simulink model "SSI_Simulator"  (R2020a)
settings: Solver=VariableStepAuto  StartTime=0.0  StopTime=10  RelTol=1e-3
values from neighbouring files (symbols this model uses):
  D = 60    [para.m]    (also in parameter.m)
  E0 = 100    [para.m]    (also in parameter.m)
  Kgov = 2    [para.m]    (also in parameter.m)
  Ki = 0.5    [para.m]    (also in parameter.m)
  Kp = 0    [para.m]    (also in parameter.m)
  KQ = 0.05    [para.m]    (also in parameter.m)
  Kvq = 1    [para.m]    (also in parameter.m)
  M = 1    [para.m]    (also in parameter.m)
  Pm = 300    [para.m]    (also in parameter.m)
  Qref = 0    [para.m]    (also in parameter.m)
  Qsig = 1    [para.m]    (also in parameter.m)
  Tgov = 0.1    [para.m]    (also in parameter.m)
  Tvq = 0.001    [para.m]    (also in parameter.m)
  Vl = 100    [para.m]    (also in parameter.m)
  Vref = 100    [para.m]    (also in parameter.m)
  wref = 2 * pi * 60    (= 376.991118431)    [para.m]    (also in parameter.m)
  Y1 = complex(G1, B1)    [para.m]    (also in parameter.m)
  Y2 = complex(G2 ,B2)    [para.m]    (also in parameter.m)
  Yg = 0    [para.m]    (also in parameter.m)
  YGG = inv(Y1 + Y2 + Yg)    [para.m]    (also in parameter.m)
undefined symbols (not defined in the file or in its folder): sw
libraries: simulink x1
settings Model: Creator=EPESL  LastModifiedBy=EPESL
settings DataIOCC: ReturnWorkspaceOutputs=off
settings DebuggingCC: AlgebraicLoopMsg=none  ArithmeticOperatorsInVariantConditions=warning
settings SFSimCC: CustomCodeUndefinedFunction=UseInterfaceOnly

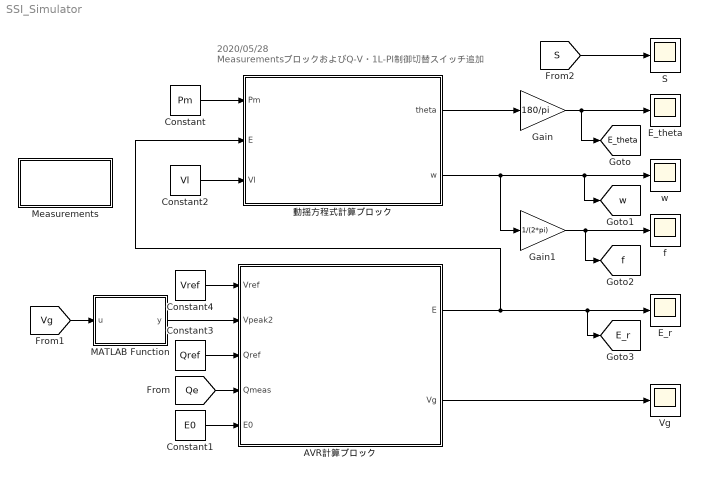
== system SSI_Simulator ==
  note: 2020/05/28
      | MeasurementsブロックおよびQ-V・1L-PI制御切替スイッチ追加
  AVR計算ブロック : Subsystem
  Constant : Constant  Value=Pm
  Constant1 : Constant  Value=E0
  Constant2 : Constant  Value=Vl
  Constant3 : Constant  Value=Qref
  Constant4 : Constant  Value=Vref
  E_r : Scope
  E_theta : Scope
  Gain : Gain  Gain=180/pi
  Gain1 : Gain  Gain=1/(2*pi)
  MATLAB Function : MATLAB Function  TreatAsAtomicUnit=on
  Measurements : Subsystem
      mask Display: color('blue');disp('Measurements')
  S : Scope
  Vg : Scope
  f : Scope
  w : Scope
  動揺方程式計算ブロック : Subsystem
  tag scope: E_r=global, E_theta=global, f=global, w=global
  wires:
  [S] -> S/1
  AVR計算ブロック/2(Vg) -> Vg/1
  MATLAB Function/1(y) -> AVR計算ブロック/2(Vpeak2)
  Constant3/1 -> AVR計算ブロック/3(Qref)
  Constant4/1 -> AVR計算ブロック/1(Vref)
  [Qe] -> AVR計算ブロック/4(Qmeas)
  [Vg] -> MATLAB Function/1(u)
  Constant/1 -> 動揺方程式計算ブロック/1(Pm)
  Constant2/1 -> 動揺方程式計算ブロック/3(Vl)
  Gain/1 -> [E_theta], E_theta/1
  動揺方程式計算ブロック/2(w) -> Gain1/1, [w], w/1
  AVR計算ブロック/1(E) -> 動揺方程式計算ブロック/2(E), [E_r], E_r/1
  Gain1/1 -> [f], f/1
  動揺方程式計算ブロック/1(theta) -> Gain/1
  Constant1/1 -> AVR計算ブロック/5(E0)

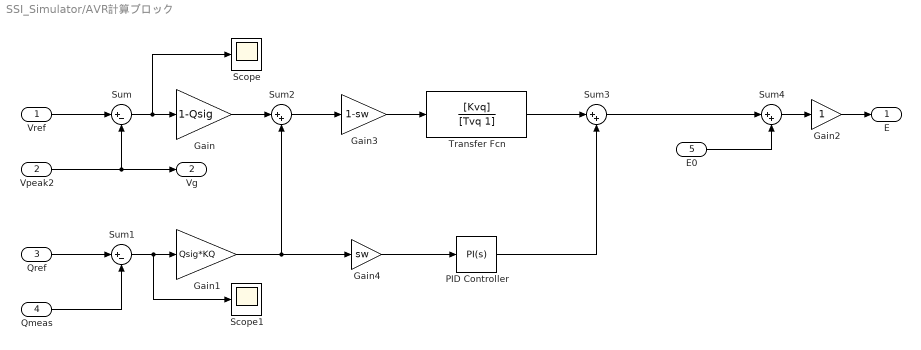
== system SSI_Simulator/AVR計算ブロック ==
  Vref : Inport
  Vpeak2 : Inport  Port=2
  Qref : Inport  Port=3
  Qmeas : Inport  Port=4
  E0 : Inport  Port=5
  Gain : Gain  Gain=1-Qsig
  Gain1 : Gain  Gain=Qsig*KQ
  Gain2 : Gain
  Gain3 : Gain  Gain=1-sw
  Gain4 : Gain  Gain=sw
  PID Controller : simulink/Continuous/PID Controller  Controller=PI  Form=Parallel  TimeDomain=Continuous-time  UseExternalTs=off  SampleTime=-1  IntegratorMethod=Forward Euler  FilterMethod=Forward Euler  ControllerParametersSource=internal  P=Kp  I=Ki  D=0  UseFilter=on  N=100  TunerSelectOption=Transfer Function Based (PID Tuner App)  InitialConditionSource=internal  InitialConditionForIntegrator=0  InitialConditionForFilter=0  DifferentiatorICPrevScaledInput=0  ExternalReset=none  TrackingMode=off  Kt=1  LimitOutput=off  UpperSaturationLimit=inf  LowerSaturationLimit=-inf  LinearizeAsGain=on  AntiWindupMode=none  Kb=1  POutMin=[]  POutMax=[]  IOutMin=[]  IOutMax=[]  DOutMin=[]  DOutMax=[]  NOutMin=[]  NOutMax=[]  SumOutMin=[]  SumOutMax=[]  SaturationOutMin=[]  SaturationOutMax=[]  PParamMin=[]  PParamMax=[]  IParamMin=[]  IParamMax=[]  DParamMin=[]  DParamMax=[]  NParamMin=[]  NParamMax=[]  KbParamMin=[]  KbParamMax=[]  KtParamMin=[]  KtParamMax=[]  KbOutMin=[]  KbOutMax=[]  KtOutMin=[]  KtOutMax=[]  IntegratorOutMin=[]  IntegratorOutMax=[]  FilterOutMin=[]  FilterOutMax=[]  SumI1OutMin=[]  SumI1OutMax=[]  SumI2OutMin=[]  SumI2OutMax=[]  SumI3OutMin=[]  SumI3OutMax=[]  SumI4OutMin=[]  SumI4OutMax=[]  SumDOutMin=[]  SumDOutMax=[]  DifferentiatorOutMin=[]  DifferentiatorOutMax=[]  FilterDiffOutCoefMin=[]  FilterDiffOutCoefMax=[]  ReciprocalOutMin=[]  ReciprocalOutMax=[]  SumDenOutMin=[]  SumDenOutMax=[]  SumNumOutMin=[]  SumNumOutMax=[]  DivideOutMin=[]  DivideOutMax=[]  UdiffTsProdOutMin=[]  UdiffTsProdOutMax=[]  NTsProdOutMin=[]  NTsProdOutMax=[]  UintegralTsProdOutMin=[]  UintegralTsProdOutMax=[]  UngainTsProdOutMin=[]  UngainTsProdOutMax=[]  IntegratorContinuousStateAttributes=''  IntegratorStateMustResolveToSignalObject=off  IntegratorRTWStateStorageClass=Auto  FilterContinuousStateAttributes=''  FilterStateMustResolveToSignalObject=off  FilterRTWStateStorageClass=Auto  ParallelPVariant=InternalParameters  IdealPVariant=Disabled  IVariant=InternalParameters  DVariant=Disabled  IntegratorVariant=Continuous  SatVariant=Disabled  AWVariant=Passthrough  PCopyVariant=Disabled  TRVariant=Disabled  FdbkBlocksVariant=Forward  IdealPFdbkVariant=Disabled  SatFdbkVariant=Disabled  DerivativeFilterVariant=Disabled  NVariant=Disabled  NCopyVariant=Disabled_SignalSpec  FilterICVariant=Disabled  IntegratorICVariant=InternalICs  ExternalResetVariant=Disabled  TRSumVariant=Passthrough  SumFdbkVariant=Disabled  SumVariant=Sum_PI  TsampFilterVariant=InternalTs  TsampNgainVariant=Passthrough  TsampIntegralVariant=Passthrough
  Scope : Scope
  Scope1 : Scope
  Sum : Sum  Inputs=|+-
  Sum1 : Sum  Inputs=|+-
  Sum2 : Sum  Inputs=|++
  Sum3 : Sum  Inputs=|++
  Sum4 : Sum  Inputs=|++
  Transfer Fcn : TransferFcn  Numerator=[Kvq]  Denominator=[Tvq 1]
  E : Outport
  Vg : Outport  Port=2
  wires:
  Transfer Fcn/1 -> Sum3/1
  Sum3/1 -> Sum4/1
  Qref/1 -> Sum1/1
  Gain1/1 -> Gain4/1, Sum2/2
  Sum4/1 -> Gain2/1
  Gain2/1 -> E/1
  PID Controller/1 -> Sum3/2
  Qmeas/1 -> Sum1/2
  Vpeak2/1 -> Vg/1, Sum/2
  Sum/1 -> Scope/1, Gain/1
  Vref/1 -> Sum/1
  Gain/1 -> Sum2/1
  Sum1/1 -> Scope1/1, Gain1/1
  Sum2/1 -> Gain3/1
  Gain3/1 -> Transfer Fcn/1
  Gain4/1 -> PID Controller/1
  E0/1 -> Sum4/2

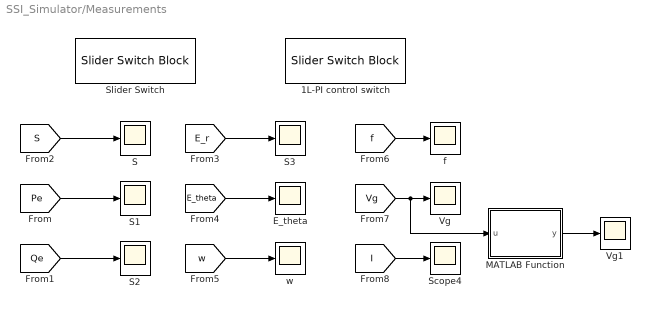
== system SSI_Simulator/Measurements ==
  1L-PI control switch : SliderSwitchBlock  LabelPosition=Hide
      settings: Values={{'1L', 'PI'}, [0 1]}
  E_theta : Scope
  MATLAB Function : MATLAB Function  TreatAsAtomicUnit=on
  S{,1..3} (4 alike) : Scope
  Scope4 : Scope
  Slider Switch : SliderSwitchBlock  LabelPosition=Hide
      settings: Values={{'Q', 'V'}, [1 0]}
  Vg : Scope
  Vg1 : Scope
  f : Scope
  w : Scope
  wires:
  [S] -> S/1
  [Pe] -> S1/1
  [Qe] -> S2/1
  [E_r] -> S3/1
  [w] -> w/1
  [I] -> Scope4/1
  [Vg] -> MATLAB Function/1(u), Vg/1
  [E_theta] -> E_theta/1
  [f] -> f/1
  MATLAB Function/1(y) -> Vg1/1

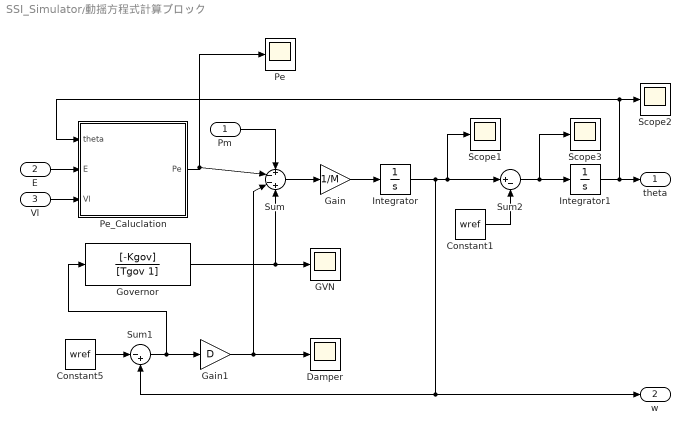
== system SSI_Simulator/動揺方程式計算ブロック ==
  Pm : Inport
  E : Inport  Port=2
  Vl : Inport  Port=3
  Constant1 : Constant  Value=wref
  Constant5 : Constant  Value=wref
  Damper : Scope
  GVN : Scope
  Gain : Gain  Gain=1/M
  Gain1 : Gain  Gain=D
  Governor : TransferFcn  Numerator=[-Kgov]  Denominator=[Tgov 1]
  Integrator : Integrator  InitialCondition=2*pi*60
  Integrator1 : Integrator
  Pe : Scope
  Pe_Caluclation : Subsystem
  Scope1 : Scope
  Scope2 : Scope
  Scope3 : Scope
  Sum : Sum  Inputs=+--+
  Sum1 : Sum  Inputs=|-+
  Sum2 : Sum  Inputs=|+-
  theta : Outport  VectorParamsAs1DForOutWhenUnconnected=off
  w : Outport  Port=2  VectorParamsAs1DForOutWhenUnconnected=off
  wires:
  Sum1/1 -> Governor/1, Gain1/1
  Gain/1 -> Integrator/1
  Constant5/1 -> Sum1/1
  Sum/1 -> Gain/1
  Gain1/1 -> Damper/1, Sum/3
  Integrator1/1 -> Pe_Caluclation/1(theta), Scope2/1, theta/1
  Pm/1 -> Sum/1
  Vl/1 -> Pe_Caluclation/3(Vl)
  Pe_Caluclation/1(Pe) -> Sum/2, Pe/1
  E/1 -> Pe_Caluclation/2(E)
  Governor/1 -> GVN/1, Sum/4
  Sum2/1 -> Scope3/1, Integrator1/1
  Integrator/1 -> Sum2/1, Scope1/1, w/1, Sum1/2
  Constant1/1 -> Sum2/2

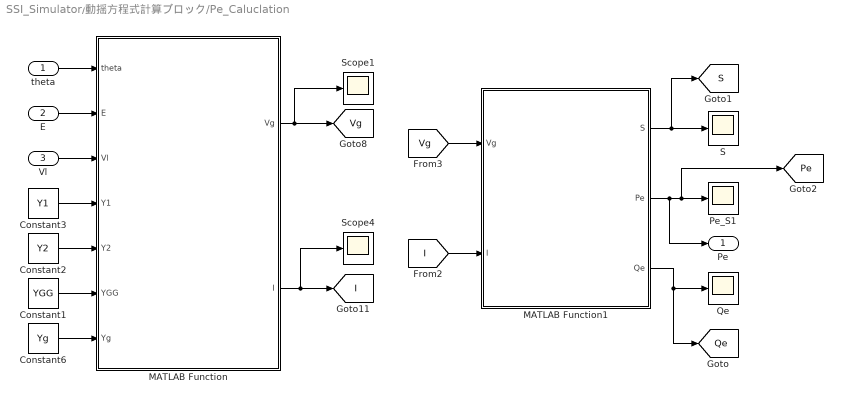
== system SSI_Simulator/動揺方程式計算ブロック/Pe_Caluclation ==
  theta : Inport
  E : Inport  Port=2
  Vl : Inport  Port=3
  Constant1 : Constant  Value=YGG
  Constant2 : Constant  Value=Y2
  Constant3 : Constant  Value=Y1
  Constant6 : Constant  Value=Yg
  MATLAB Function : MATLAB Function  TreatAsAtomicUnit=on
  MATLAB Function1 : MATLAB Function  TreatAsAtomicUnit=on
  Pe_S1 : Scope
  Qe : Scope
  S : Scope
  Scope1 : Scope
  Scope4 : Scope
  Pe : Outport
  tag scope: I=global, Pe=global, Qe=global, S=global, Vg=global
  wires:
  MATLAB Function/1(Vg) -> Scope1/1, [Vg]
  MATLAB Function1/1(S) -> [S], S/1
  [I] -> MATLAB Function1/2(I)
  [Vg] -> MATLAB Function1/1(Vg)
  MATLAB Function/2(I) -> Scope4/1, [I]
  Constant6/1 -> MATLAB Function/7(Yg)
  Constant3/1 -> MATLAB Function/4(Y1)
  MATLAB Function1/2(Pe) -> Pe/1, [Pe], Pe_S1/1
  MATLAB Function1/3(Qe) -> [Qe], Qe/1
  Vl/1 -> MATLAB Function/3(Vl)
  E/1 -> MATLAB Function/2(E)
  theta/1 -> MATLAB Function/1(theta)
  Constant2/1 -> MATLAB Function/5(Y2)
  Constant1/1 -> MATLAB Function/6(YGG)

== matlab function SSI_Simulator/動揺方程式計算ブロック/Pe_Caluclation/MATLAB Function1 ==
  data: Vg input; S output; I input; Pe output; Qe output
function [S, Pe, Qe]  = Func(Vg, I)

S = conj(Vg) .* I;  % 進相条件
Pe = real(S);
Qe = imag(S);

== matlab function SSI_Simulator/動揺方程式計算ブロック/Pe_Caluclation/MATLAB Function ==
  data: theta input; Vg output; E input; I output; Vl input; Y1 input; Y2 input; YGG input; Yg input
function [Vg, I]= Func(theta, E, Vl, Y1, Y2, YGG, Yg)

Ea = E * exp(1i * theta);

Vg = (YGG) * ((Y1 * Ea) + (Y2 * Vl));
I = Y1 * Ea - Y1 * Vg;

== matlab function SSI_Simulator/MATLAB Function ==
  data: u input; y output
function y = Real(u)

y = real(u);

== matlab function SSI_Simulator/Measurements/MATLAB Function ==
  data: u input; y output
function y = Real(u)

y = real(u);
